simulink model "requirementsTable"  (R2022a)
settings: Solver=VariableStepAuto  StartTime=0.0  StopTime=10.0  RelTol=1e-3
settings Model: Creator=bryan  LastModifiedBy=bryan

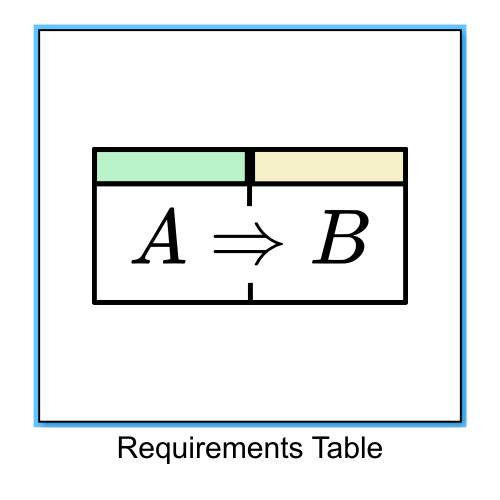
[thumbnail: Simulink's stored preview of the top-level diagram]
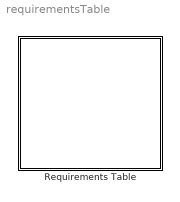
== system requirementsTable ==
  Requirements Table : Requirements Table  TreatAsAtomicUnit=on

== stateflow chart requirementsTable/Requirements Table ==
  (default) -> (junction 1073741860)
  (junction 1073741860) -> (junction 1073741861) : {
      | % SF_REQ_REV_07
      | }
  (junction 1073741861) -> (junction 1073741863) : {
      | % HEADER_ASSIGNMENTS
      |
      | }
  (junction 1073741863) -> (junction 1073741865) : {
      | % START_A_4
      | }
  (junction 1073741865) -> (junction 1073741867) : {
      | }
  (junction 1073741867) -> (junction 1073741869)
  (junction 1073741869) -> (junction 1073741871) : {
      | }
  (junction 1073741871) -> (junction 1073741873) : {
      | % END_A_4
      | }
  (junction 1073741873) -> (junction 1073741910) : {
      | % START_R_1
      | }
  (junction 1073741910) -> (junction 1073741912) : {
      | }
  (junction 1073741912) -> (junction 1073741914) : {
      |
      |
      | }
  (junction 1073741914) -> (junction 1073741916) : {
      | }
  (junction 1073741916) -> (junction 1073741932) : {
      | % START_R_7
      | }
  (junction 1073741932) -> (junction 1073741934) : {
      | }
  (junction 1073741934) -> (junction 1073741936) : {
      |
      |
      | }
  (junction 1073741936) -> (junction 1073741938) : {
      | }
  (junction 1073741938) -> (junction 1073741990) : {
      | % START_R_10
      | }
  (junction 1073741990) -> (junction 1073741992) : {
      | }
  (junction 1073741992) -> (junction 1073741994)
  (junction 1073741994) -> (junction 1073741996) [order 1] : [(MODE == 0 || after(ATR_REFACTORY_PERIOD, msec))]
  (junction 1073741994) -> (junction 1073742002) [order 2]
  (junction 1073741996) -> (junction 1073741998) : {
      | reqtable_postcondition((ATR_PACE_CTRL == false), 'R:1.1.1');
      |
      |
      | }
  (junction 1073741998) -> (junction 1073742000) : {
      | }
  (junction 1073742000) -> (junction 1073742002)
  (junction 1073742002) -> (junction 1073742004)
  (junction 1073742004) -> (junction 1073742006) : {
      | % END_R_10
      | }
  (junction 1073742006) -> (junction 1073742011) : {
      | % START_R_13
      | }
  (junction 1073742011) -> (junction 1073742013) : {
      | }
  (junction 1073742013) -> (junction 1073742015)
  (junction 1073742015) -> (junction 1073742017) [order 1] : [(MODE == 0 || after(ATR_REFACTORY_PERIOD, msec))]
  (junction 1073742015) -> (junction 1073742023) [order 2]
  (junction 1073742017) -> (junction 1073742019) : {
      | reqtable_postcondition((VENT_PACE_CTRL == false), 'R:1.1.2');
      |
      |
      | }
  (junction 1073742019) -> (junction 1073742021) : {
      | }
  (junction 1073742021) -> (junction 1073742023)
  (junction 1073742023) -> (junction 1073742025)
  (junction 1073742025) -> (junction 1073742027) : {
      | % END_R_13
      | }
  (junction 1073742027) -> (junction 1073742032) : {
      | % START_R_16
      | }
  (junction 1073742032) -> (junction 1073742034) : {
      | }
  (junction 1073742034) -> (junction 1073742036)
  (junction 1073742036) -> (junction 1073742038) [order 1] : [(MODE == 0 || after(ATR_REFACTORY_PERIOD, msec))]
  (junction 1073742036) -> (junction 1073742044) [order 2]
  (junction 1073742038) -> (junction 1073742040) : {
      | reqtable_postcondition((PACING_REF_PWM == ATR_AMPLITUDE), 'R:1.1.3');
      |
      |
      | }
  (junction 1073742040) -> (junction 1073742042) : {
      | }
  (junction 1073742042) -> (junction 1073742044)
  (junction 1073742044) -> (junction 1073742046)
  (junction 1073742046) -> (junction 1073742048) : {
      | % END_R_16
      | }
  (junction 1073742048) -> (junction 1073742053) : {
      | % START_R_19
      | }
  (junction 1073742053) -> (junction 1073742055) : {
      | }
  (junction 1073742055) -> (junction 1073742057)
  (junction 1073742057) -> (junction 1073742059) [order 1] : [(MODE == 0 || after(ATR_REFACTORY_PERIOD, msec))]
  (junction 1073742057) -> (junction 1073742065) [order 2]
  (junction 1073742059) -> (junction 1073742061) : {
      | reqtable_postcondition((PACE_CHARGE_CTRL == true), 'R:1.1.4');
      |
      |
      | }
  (junction 1073742061) -> (junction 1073742063) : {
      | }
  (junction 1073742063) -> (junction 1073742065)
  (junction 1073742065) -> (junction 1073742067)
  (junction 1073742067) -> (junction 1073742069) : {
      | % END_R_19
      | }
  (junction 1073742069) -> (junction 1073742144) : {
      | % START_R_22
      | }
  (junction 1073742144) -> (junction 1073742146) : {
      | }
  (junction 1073742146) -> (junction 1073742148)
  (junction 1073742148) -> (junction 1073742150) [order 1] : [(MODE == 0 || after(ATR_REFACTORY_PERIOD, msec))]
  (junction 1073742148) -> (junction 1073742156) [order 2]
  (junction 1073742150) -> (junction 1073742152) : {
      | reqtable_postcondition((PACE_GND_CTRL == true), 'R:1.1.5');
      |
      |
      | }
  (junction 1073742152) -> (junction 1073742154) : {
      | }
  (junction 1073742154) -> (junction 1073742156)
  (junction 1073742156) -> (junction 1073742158)
  (junction 1073742158) -> (junction 1073742160) : {
      | % END_R_22
      | }
  (junction 1073742160) -> (junction 1073742165) : {
      | % START_R_25
      | }
  (junction 1073742165) -> (junction 1073742167) : {
      | }
  (junction 1073742167) -> (junction 1073742169)
  (junction 1073742169) -> (junction 1073742171) [order 1] : [(MODE == 0 || after(ATR_REFACTORY_PERIOD, msec))]
  (junction 1073742169) -> (junction 1073742177) [order 2]
  (junction 1073742171) -> (junction 1073742173) : {
      | reqtable_postcondition((Z_ATR_CTRL == false), 'R:1.1.6');
      |
      |
      | }
  (junction 1073742173) -> (junction 1073742175) : {
      | }
  (junction 1073742175) -> (junction 1073742177)
  (junction 1073742177) -> (junction 1073742179)
  (junction 1073742179) -> (junction 1073742181) : {
      | % END_R_25
      | }
  (junction 1073742181) -> (junction 1073742231) : {
      | % START_R_34
      | }
  (junction 1073742231) -> (junction 1073742233) : {
      | }
  (junction 1073742233) -> (junction 1073742235)
  (junction 1073742235) -> (junction 1073742237) [order 1] : [(MODE == 0 || after(ATR_REFACTORY_PERIOD, msec))]
  (junction 1073742235) -> (junction 1073742243) [order 2]
  (junction 1073742237) -> (junction 1073742239) : {
      | reqtable_postcondition((Z_VENT_CTRL == false), 'R:1.1.7');
      |
      |
      | }
  (junction 1073742239) -> (junction 1073742241) : {
      | }
  (junction 1073742241) -> (junction 1073742243)
  (junction 1073742243) -> (junction 1073742245)
  (junction 1073742245) -> (junction 1073742247) : {
      | % END_R_34
      | }
  (junction 1073742247) -> (junction 1073742252) : {
      | % START_R_37
      | }
  (junction 1073742252) -> (junction 1073742254) : {
      | }
  (junction 1073742254) -> (junction 1073742256)
  (junction 1073742256) -> (junction 1073742258) [order 1] : [(MODE == 0 || after(ATR_REFACTORY_PERIOD, msec))]
  (junction 1073742256) -> (junction 1073742264) [order 2]
  (junction 1073742258) -> (junction 1073742260) : {
      | reqtable_postcondition((VENT_GND_CTRL == false), 'R:1.1.8');
      |
      |
      | }
  (junction 1073742260) -> (junction 1073742262) : {
      | }
  (junction 1073742262) -> (junction 1073742264)
  (junction 1073742264) -> (junction 1073742266)
  (junction 1073742266) -> (junction 1073742268) : {
      | % END_R_37
      | }
  (junction 1073742268) -> (junction 1073742186) : {
      | % START_R_31
      | }
  (junction 1073742186) -> (junction 1073742188) : {
      | }
  (junction 1073742188) -> (junction 1073742190)
  (junction 1073742190) -> (junction 1073742192) [order 1] : [(MODE == 0 || after(ATR_REFACTORY_PERIOD, msec))]
  (junction 1073742190) -> (junction 1073742198) [order 2]
  (junction 1073742192) -> (junction 1073742194) : {
      | reqtable_postcondition((ATR_GND_CTRL == true), 'R:1.1.9');
      |
      |
      | }
  (junction 1073742194) -> (junction 1073742196) : {
      | }
  (junction 1073742196) -> (junction 1073742198)
  (junction 1073742198) -> (junction 1073742200)
  (junction 1073742200) -> (junction 1073742981) : {
      | % END_R_31
      | }
  (junction 1073742981) -> (junction 1073742297) : {
      | % START_R_43
      | }
  (junction 1073742297) -> (junction 1073742299) : {
      | }
  (junction 1073742299) -> (junction 1073742301)
  (junction 1073742301) -> (junction 1073742303) [order 1] : [(MODE == 0 || after(ATR_REFACTORY_PERIOD, msec))]
  (junction 1073742301) -> (junction 1073742309) [order 2]
  (junction 1073742303) -> (junction 1073742305) : {
      | reqtable_postcondition((RED_LED == false), 'R:1.1.10');
      |
      |
      | }
  (junction 1073742305) -> (junction 1073742307) : {
      | }
  (junction 1073742307) -> (junction 1073742309)
  (junction 1073742309) -> (junction 1073742311)
  (junction 1073742311) -> (junction 1073742313) : {
      | % END_R_43
      | }
  (junction 1073742313) -> (junction 1073742318) : {
      | % START_R_40
      | }
  (junction 1073742318) -> (junction 1073742320) : {
      | }
  (junction 1073742320) -> (junction 1073742322)
  (junction 1073742322) -> (junction 1073742324) [order 1] : [(MODE == 0 || after(ATR_REFACTORY_PERIOD, msec))]
  (junction 1073742322) -> (junction 1073742330) [order 2]
  (junction 1073742324) -> (junction 1073742326) : {
      | reqtable_postcondition((BLUE_LED == false), 'R:1.1.11');
      |
      |
      | }
  (junction 1073742326) -> (junction 1073742328) : {
      | }
  (junction 1073742328) -> (junction 1073742330)
  (junction 1073742330) -> (junction 1073742332)
  (junction 1073742332) -> (junction 1073742334) : {
      | % END_R_40
      | }
  (junction 1073742334) -> (junction 1073742351) : {
      | % START_R_46
      | }
  (junction 1073742351) -> (junction 1073742353) : {
      | }
  (junction 1073742353) -> (junction 1073742355)
  (junction 1073742355) -> (junction 1073742357) [order 1] : [(MODE == 0 || after(ATR_REFACTORY_PERIOD, msec))]
  (junction 1073742355) -> (junction 1073742363) [order 2]
  (junction 1073742357) -> (junction 1073742359) : {
      | reqtable_postcondition((GREEN_LED == false), 'R:1.1.12');
      |
      |
      | }
  (junction 1073742359) -> (junction 1073742361) : {
      | }
  (junction 1073742361) -> (junction 1073742363)
  (junction 1073742363) -> (junction 1073742365)
  (junction 1073742365) -> (junction 1073743060) : {
      | % END_R_46
      | }
  (junction 1073743060) -> (junction 1073741950) : {
      | % END_R_7
      | }
  (junction 1073741950) -> (junction 1073742384) : {
      | % START_R_49
      | }
  (junction 1073742384) -> (junction 1073742386) : {
      | }
  (junction 1073742386) -> (junction 1073742388) : {
      |
      |
      | }
  (junction 1073742388) -> (junction 1073742390) : {
      | }
  (junction 1073742390) -> (junction 1073742544) : {
      | % START_R_52
      | }
  (junction 1073742544) -> (junction 1073742546) : {
      | }
  (junction 1073742546) -> (junction 1073742548)
  (junction 1073742548) -> (junction 1073742550) [order 1] : [(MODE == 1 && ATR_CMP_DETECT)]
  (junction 1073742548) -> (junction 1073742556) [order 2]
  (junction 1073742550) -> (junction 1073742552) : {
      | reqtable_postcondition((GREEN_LED == true), 'R:1.2.1');
      |
      |
      | }
  (junction 1073742552) -> (junction 1073742554) : {
      | }
  (junction 1073742554) -> (junction 1073742556)
  (junction 1073742556) -> (junction 1073742558)
  (junction 1073742558) -> (junction 1073742414) : {
      | % END_R_52
      | }
  (junction 1073742414) -> (junction 1073742932) : {
      | % START_R_103
      | }
  (junction 1073742932) -> (junction 1073742934) : {
      | }
  (junction 1073742934) -> (junction 1073742936)
  (junction 1073742936) -> (junction 1073742938) [order 1] : [(MODE == 1 && ATR_CMP_DETECT)]
  (junction 1073742936) -> (junction 1073742944) [order 2]
  (junction 1073742938) -> (junction 1073742940) : {
      | reqtable_postcondition((ATR_Delta == 0), 'R:1.2.2');
      |
      |
      | }
  (junction 1073742940) -> (junction 1073742942) : {
      | }
  (junction 1073742942) -> (junction 1073742944)
  (junction 1073742944) -> (junction 1073742946)
  (junction 1073742946) -> (junction 1073742948) : {
      | % END_R_103
      | }
  (junction 1073742948) -> (junction 1073742998) : {
      | % START_R_109
      | }
  (junction 1073742998) -> (junction 1073743000) : {
      | }
  (junction 1073743000) -> (junction 1073743002)
  (junction 1073743002) -> (junction 1073743004) [order 1] : [(MODE == 1 && ATR_CMP_DETECT && after(ATR_REFACTORY_PERIOD, msec))]
  (junction 1073743002) -> (junction 1073743010) [order 2]
  (junction 1073743004) -> (junction 1073743006) : {
      | reqtable_postcondition((ATR_Delta == ATR_Delta + ATR_REFACTORY_PERIOD), 'R:1.2.3');
      |
      |
      | }
  (junction 1073743006) -> (junction 1073743008) : {
      | }
  (junction 1073743008) -> (junction 1073743010)
  (junction 1073743010) -> (junction 1073743012)
  (junction 1073743012) -> (junction 1073743014) : {
      | % END_R_109
      | }
  (junction 1073743014) -> (junction 1073742402) : {
      | % END_R_49
      | }
  (junction 1073742402) -> (junction 1073742613) : {
      | % START_R_67
      | }
  (junction 1073742613) -> (junction 1073742615) : {
      | }
  (junction 1073742615) -> (junction 1073742617) : {
      |
      |
      | }
  (junction 1073742617) -> (junction 1073742619) : {
      | }
  (junction 1073742619) -> (junction 1073742695) : {
      | % START_R_76
      | }
  (junction 1073742695) -> (junction 1073742697) : {
      | }
  (junction 1073742697) -> (junction 1073742699)
  (junction 1073742699) -> (junction 1073742701) [order 1] : [(after([60000/LOWER_RATE_LIMIT] - ATR_Delta, msec))]
  (junction 1073742699) -> (junction 1073742707) [order 2]
  (junction 1073742701) -> (junction 1073742703) : {
      | reqtable_postcondition((PACE_CHARGE_CTRL == false), 'R:1.3.1');
      |
      |
      | }
  (junction 1073742703) -> (junction 1073742705) : {
      | }
  (junction 1073742705) -> (junction 1073742707)
  (junction 1073742707) -> (junction 1073742709)
  (junction 1073742709) -> (junction 1073742711) : {
      | % END_R_76
      | }
  (junction 1073742711) -> (junction 1073742716) : {
      | % START_R_79
      | }
  (junction 1073742716) -> (junction 1073742718) : {
      | }
  (junction 1073742718) -> (junction 1073742720)
  (junction 1073742720) -> (junction 1073742722) [order 1] : [(after([60000/LOWER_RATE_LIMIT] - ATR_Delta, msec))]
  (junction 1073742720) -> (junction 1073742728) [order 2]
  (junction 1073742722) -> (junction 1073742724) : {
      | reqtable_postcondition((PACE_GND_CTRL == true), 'R:1.3.2');
      |
      |
      | }
  (junction 1073742724) -> (junction 1073742726) : {
      | }
  (junction 1073742726) -> (junction 1073742728)
  (junction 1073742728) -> (junction 1073742730)
  (junction 1073742730) -> (junction 1073742732) : {
      | % END_R_79
      | }
  (junction 1073742732) -> (junction 1073742737) : {
      | % START_R_82
      | }
  (junction 1073742737) -> (junction 1073742739) : {
      | }
  (junction 1073742739) -> (junction 1073742741)
  (junction 1073742741) -> (junction 1073742743) [order 1] : [(after([60000/LOWER_RATE_LIMIT] - ATR_Delta, msec))]
  (junction 1073742741) -> (junction 1073742749) [order 2]
  (junction 1073742743) -> (junction 1073742745) : {
      | reqtable_postcondition((VENT_PACE_CTRL == false), 'R:1.3.3');
      |
      |
      | }
  (junction 1073742745) -> (junction 1073742747) : {
      | }
  (junction 1073742747) -> (junction 1073742749)
  (junction 1073742749) -> (junction 1073742751)
  (junction 1073742751) -> (junction 1073742753) : {
      | % END_R_82
      | }
  (junction 1073742753) -> (junction 1073742758) : {
      | % START_R_85
      | }
  (junction 1073742758) -> (junction 1073742760) : {
      | }
  (junction 1073742760) -> (junction 1073742762)
  (junction 1073742762) -> (junction 1073742764) [order 1] : [(after([60000/LOWER_RATE_LIMIT] - ATR_Delta, msec))]
  (junction 1073742762) -> (junction 1073742770) [order 2]
  (junction 1073742764) -> (junction 1073742766) : {
      | reqtable_postcondition((VENT_GND_CTRL == false), 'R:1.3.4');
      |
      |
      | }
  (junction 1073742766) -> (junction 1073742768) : {
      | }
  (junction 1073742768) -> (junction 1073742770)
  (junction 1073742770) -> (junction 1073742772)
  (junction 1073742772) -> (junction 1073742774) : {
      | % END_R_85
      | }
  (junction 1073742774) -> (junction 1073742779) : {
      | % START_R_88
      | }
  (junction 1073742779) -> (junction 1073742781) : {
      | }
  (junction 1073742781) -> (junction 1073742783)
  (junction 1073742783) -> (junction 1073742785) [order 1] : [(after([60000/LOWER_RATE_LIMIT] - ATR_Delta, msec))]
  (junction 1073742783) -> (junction 1073742791) [order 2]
  (junction 1073742785) -> (junction 1073742787) : {
      | reqtable_postcondition((Z_ATR_CTRL == false), 'R:1.3.5');
      |
      |
      | }
  (junction 1073742787) -> (junction 1073742789) : {
      | }
  (junction 1073742789) -> (junction 1073742791)
  (junction 1073742791) -> (junction 1073742793)
  (junction 1073742793) -> (junction 1073742795) : {
      | % END_R_88
      | }
  (junction 1073742795) -> (junction 1073742800) : {
      | % START_R_91
      | }
  (junction 1073742800) -> (junction 1073742802) : {
      | }
  (junction 1073742802) -> (junction 1073742804)
  (junction 1073742804) -> (junction 1073742806) [order 1] : [(after([60000/LOWER_RATE_LIMIT] - ATR_Delta, msec))]
  (junction 1073742804) -> (junction 1073742812) [order 2]
  (junction 1073742806) -> (junction 1073742808) : {
      | reqtable_postcondition((Z_VENT_CTRL == false), 'R:1.3.6');
      |
      |
      | }
  (junction 1073742808) -> (junction 1073742810) : {
      | }
  (junction 1073742810) -> (junction 1073742812)
  (junction 1073742812) -> (junction 1073742814)
  (junction 1073742814) -> (junction 1073742816) : {
      | % END_R_91
      | }
  (junction 1073742816) -> (junction 1073742857) : {
      | % START_R_94
      | }
  (junction 1073742857) -> (junction 1073742859) : {
      | }
  (junction 1073742859) -> (junction 1073742861)
  (junction 1073742861) -> (junction 1073742863) [order 1] : [(after([60000/LOWER_RATE_LIMIT] - ATR_Delta, msec))]
  (junction 1073742861) -> (junction 1073742869) [order 2]
  (junction 1073742863) -> (junction 1073742865) : {
      | reqtable_postcondition((ATR_GND_CTRL == false), 'R:1.3.7');
      |
      |
      | }
  (junction 1073742865) -> (junction 1073742867) : {
      | }
  (junction 1073742867) -> (junction 1073742869)
  (junction 1073742869) -> (junction 1073742871)
  (junction 1073742871) -> (junction 1073742873) : {
      | % END_R_94
      | }
  (junction 1073742873) -> (junction 1073742878) : {
      | % START_R_97
      | }
  (junction 1073742878) -> (junction 1073742880) : {
      | }
  (junction 1073742880) -> (junction 1073742882)
  (junction 1073742882) -> (junction 1073742884) [order 1] : [(after([60000/LOWER_RATE_LIMIT] - ATR_Delta, msec))]
  (junction 1073742882) -> (junction 1073742890) [order 2]
  (junction 1073742884) -> (junction 1073742886) : {
      | reqtable_postcondition((ATR_PACE_CTRL == true), 'R:1.3.8');
      |
      |
      | }
  (junction 1073742886) -> (junction 1073742888) : {
      | }
  (junction 1073742888) -> (junction 1073742890)
  (junction 1073742890) -> (junction 1073742892)
  (junction 1073742892) -> (junction 1073742894) : {
      | % END_R_97
      | }
  (junction 1073742894) -> (junction 1073742899) : {
      | % START_R_100
      | }
  (junction 1073742899) -> (junction 1073742901) : {
      | }
  (junction 1073742901) -> (junction 1073742903)
  (junction 1073742903) -> (junction 1073742905) [order 1] : [(after([60000/LOWER_RATE_LIMIT] - ATR_Delta, msec))]
  (junction 1073742903) -> (junction 1073742911) [order 2]
  (junction 1073742905) -> (junction 1073742907) : {
      | reqtable_postcondition((RED_LED == true), 'R:1.3.9');
      |
      |
      | }
  (junction 1073742907) -> (junction 1073742909) : {
      | }
  (junction 1073742909) -> (junction 1073742911)
  (junction 1073742911) -> (junction 1073742913)
  (junction 1073742913) -> (junction 1073742915) : {
      | % END_R_100
      | }
  (junction 1073742915) -> (junction 1073743031) : {
      | % START_R_112
      | }
  (junction 1073743031) -> (junction 1073743033) : {
      | }
  (junction 1073743033) -> (junction 1073743035)
  (junction 1073743035) -> (junction 1073743037) [order 1] : [(after([60000/LOWER_RATE_LIMIT] - ATR_Delta, msec) && after(ATR_PULSE_WIDTH, msec))]
  (junction 1073743035) -> (junction 1073743043) [order 2]
  (junction 1073743037) -> (junction 1073743039) : {
      | reqtable_postcondition((ATR_Delta == ATR_PULSE_WIDTH), 'R:1.3.10');
      |
      |
      | }
  (junction 1073743039) -> (junction 1073743041) : {
      | }
  (junction 1073743041) -> (junction 1073743043)
  (junction 1073743043) -> (junction 1073743045)
  (junction 1073743045) -> (junction 1073743047) : {
      | % END_R_112
      | }
  (junction 1073743047) -> (junction 1073742631) : {
      | % END_R_67
      | }
  (junction 1073742631) -> (junction 1073741928) : {
      | % END_R_1
      | }
